simulink model "localization"  (R2025a)
settings: Solver=ode1  StartTime=0.0  StopTime=inf  FixedStep=1/60  RelTol=1e-3  EnableMultiTasking=on
model workspace (MAT data in the model file):
  downCamStepSize = Simulink.Parameter
  downCamStepSize.Value = Simulink.data.Expression
  downCamStepSize.Value.ExpressionString = "qc_get_step_size*ceil(1/60/qc_get_step_size)"
  downCamStepSize.Complexity = 'real'
  downCamStepSize.Dimensions = -1
  downCamStepSize.DataType = 'auto'
  lidarStepSize = Simulink.Parameter
  lidarStepSize.Value = Simulink.data.Expression
  lidarStepSize.Value.ExpressionString = "qc_get_step_size*ceil(1/5/qc_get_step_size)"
  lidarStepSize.Complexity = 'real'
  lidarStepSize.Dimensions = -1
  lidarStepSize.DataType = 'auto'
  mainStepSize = Simulink.Parameter
  mainStepSize.Value = Simulink.data.Expression
  mainStepSize.Value.ExpressionString = "qc_get_step_size"
  mainStepSize.Complexity = 'real'
  mainStepSize.Dimensions = -1
  mainStepSize.DataType = 'auto'
  mode = Simulink.Parameter
  mode.Value = 1
  mode.Complexity = 'real'
  mode.Dimensions = [1 1]
  mode.Description = '0 - education speeds via wheel speed commands
    | 1 - education speeds via body speed commands
    | 2 - research speeds via wheel speed commands
    | 3 - research speeds via body speed commands'
  mode.DataType = 'auto'
  realSenseStepSize = Simulink.Parameter
  realSenseStepSize.Value = Simulink.data.Expression
  realSenseStepSize.Value.ExpressionString = "qc_get_step_size*ceil(1/30/qc_get_step_size)"
  realSenseStepSize.Complexity = 'real'
  realSenseStepSize.Dimensions = -1
  realSenseStepSize.DataType = 'auto'
undefined symbols (not defined in the file): Point
libraries: quarc_library x17, simulink x1
settings Model: SimulationMode=external  ExtModeTrigDuration=10000  Creator=mbohra  LastModifiedBy=rdu
settings SolverCC: AlgebraicLoopSolver=TrustRegion  PositivePriorityOrder=on
settings DataIOCC: ReturnWorkspaceOutputs=off
settings DebuggingCC: ParameterPrecisionLossMsg=none  UnconnectedInputMsg=warning  UnconnectedOutputMsg=warning  UnconnectedLineMsg=warning  ArithmeticOperatorsInVariantConditions=warning
settings HardwareCC: ProdBitPerLong=64.0  ProdLargestAtomicInteger=LongLong  ProdLargestAtomicFloat=Double  ProdLongLongMode=on  ProdHWDeviceType=ARM Compatible->ARM 64-bit (LP64)
settings ModelReferenceCC: EnableRefExpFcnMdlSchedulingChecks=on
settings SFSimCC: SimUseLocalCustomCode=off  CustomCodeUndefinedFunction=UseInterfaceOnly
settings RTWCC: SystemTargetFile=quarc_linux_qbot_platform.tlc  TemplateMakefile=quarc_default_tmf  RTWUseLocalCustomCode=off  Toolchain=QUARC linux_qbot_platform | gmake (64-bit Windows)  BuildConfiguration=Faster Runs  GPUComputeCapability=3.5  Description=QUARC Linux QBot Platform Target Using Toolchain
settings CodeAppCC: StateflowObjectComments=on
settings STFCustomTargetCC: SystemTargetFile=quarc_linux_qbot_platform.tlc  TargetLangStandard=C99 (ISO)  MultiwordLength=2048.0  DynamicStringBufferSize=256.0  ConcurrentExecutionCompliant=on  UseToolchainInfoCompliant=on  MinimumThreadPriority=20.0  StripSymbols=off
settings GRTTargetCC: ExtMode=on  ExtModeMexFile=quarc_comm  ExtModeMexArgs='-w -d /tmp -uri %u','tcpip://192.168.5.4:17001'  ParMdlRefBuildCompliant=off  CompOptLevelCompliant=off  CombineOutputUpdateFcns=off  MatFileLogging=off  CPPClassGenCompliant=off  GRTInterface=on
settings ConfigComp: CovMetricSettings=dswe

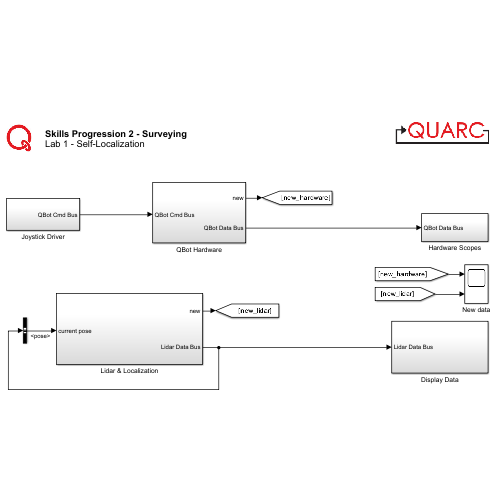
[thumbnail: Simulink's stored preview of the top-level diagram]
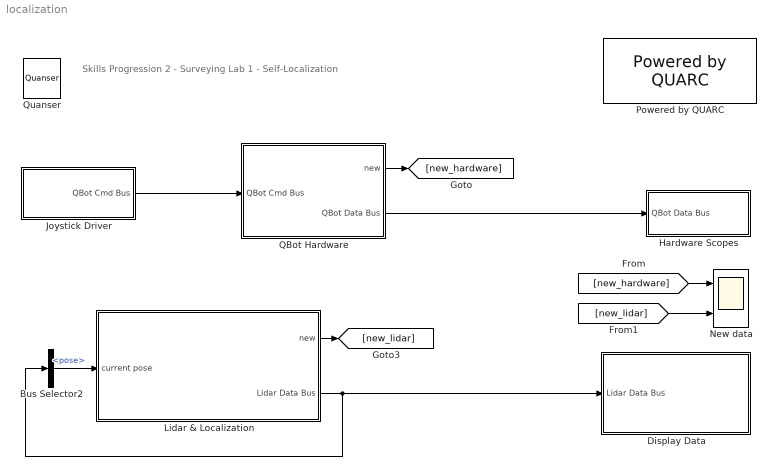
== system localization ==
  note: Skills Progression 2 - Surveying
      | Lab 1 - Self-Localization
  Bus Selector2 : BusSelector  OutputSignals=pose
  Display Data : Subsystem
  Hardware Scopes : Subsystem
  Joystick Driver : Subsystem
  Lidar & Localization : Subsystem
  New data : Scope  NumInputPorts=2
      settings: Title=Hardware Data New?  ActiveDisplayYMinimum=0.9  ActiveDisplayYMaximum=1.1  DataLoggingDecimation=10  DataLoggingVariableName=ScopeData2
  Powered by QUARC : quarc_library/Logos/Powered by QUARC
  QBot Hardware : Subsystem
  Quanser : quarc_library/Logos/Quanser
  wires:
  QBot Hardware/1(new) -> [new_hardware]
  Lidar & Localization/1(new) -> [new_lidar]
  [new_lidar] -> New data/2
  [new_hardware] -> New data/1
  Bus Selector2/1 -> Lidar & Localization/1(current pose)  "<pose>"
  Lidar & Localization/2(Lidar Data Bus) -> Bus Selector2/1, Display Data/1(Lidar Data Bus)
  Joystick Driver/1(QBot Cmd Bus) -> QBot Hardware/1(QBot Cmd Bus)
  QBot Hardware/2(QBot Data Bus) -> Hardware Scopes/1(QBot Data Bus)

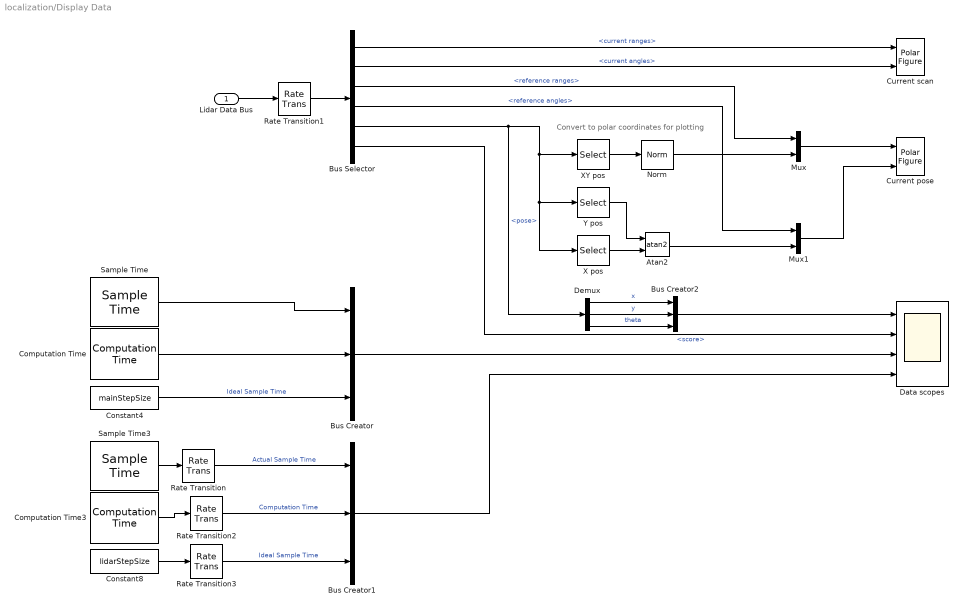
== system localization/Display Data ==
  note: Convert to polar coordinates for plotting
  Lidar Data Bus : Inport
  Atan2 : Trigonometry  Operator=atan2
  Bus Creator : BusCreator  Inputs=3
  Bus Creator1 : BusCreator  Inputs=3
  Bus Creator2 : BusCreator  Inputs=3
  Bus Selector : BusSelector  OutputSignals=current ranges,current angles,reference ranges,reference angles,pose,score
  Computation Time : quarc_library/Sources/Time/Computation Time  sample_time=mainStepSize  use_model=on  use_cpu_time=off
  Computation Time3 : quarc_library/Sources/Time/Computation Time  sample_time=lidarStepSize  use_model=on  use_cpu_time=off
  Constant4 : Constant  Value=mainStepSize
  Constant8 : Constant  Value=lidarStepSize
  Current pose : quarc_library/Sinks/Figures/Polar Figure  figure_mode=Use figure window  figure_tag=figure1  axes_tag=axes1  plot_mode=Frame-based  minimum_rho=0  maximum_rho=4  minimum_theta=0  maximum_theta=360  zero_location=right  direction=counterclockwise  buffer_size=421  update_rate=1  sample_time=-1  initial_position="875  207  831  654"  initial_visibility=off  line1_style=None  line1_width=0.5  line1_color=[1 0 0]  marker1=Point (.)  marker1_size=6  marker1_edge_color=[1 0 0]  marker1_face_color=[1 0 0]  line2_style=None  line2_width=0.5  line2_color=[0.85098 0.32549 0.0980392]  marker2=Cross (x)  marker2_size=6  marker2_edge_color=[0.85098 0.32549 0.0980392]  marker2_face_color=[0.85098 0.32549 0.0980392]  line3_style=Solid line (-)  line3_width=0.5  line3_color=[0.929412 0.694118 0.12549]  marker3=None  marker3_size=6  marker3_edge_color=[0.929412 0.694118 0.12549]  marker3_face_color=[0.929412 0.694118 0.12549]  line4_style=Solid line (-)  line4_width=0.5  line4_color=[0.494118 0.184314 0.556863]  marker4=None  marker4_size=6  marker4_edge_color=[0.494118 0.184314 0.556863]  marker4_face_color=[0.494118 0.184314 0.556863]  line5_style=Solid line (-)  line5_width=0.5  line5_color=[0.466667 0.67451 0.188235]  marker5=None  marker5_size=6  marker5_edge_color=[0.466667 0.67451 0.188235]  marker5_face_color=[0.466667 0.67451 0.188235]
      settings: SourceProductName=QUARC Targets
  Current scan : quarc_library/Sinks/Figures/Polar Figure  figure_mode=Use figure window  figure_tag=figure1  axes_tag=axes1  plot_mode=Frame-based  minimum_rho=0  maximum_rho=4  minimum_theta=0  maximum_theta=360  zero_location=right  direction=counterclockwise  buffer_size=2  update_rate=1  sample_time=-1  initial_position="60    84  1189   906"  initial_visibility=off  line1_style=None  line1_width=0.5  line1_color=[1 0 0]  marker1=Point (.)  marker1_size=6  marker1_edge_color=[1 0 0]  marker1_face_color=[1 0 0]  line2_style=Solid line (-)  line2_width=0.5  line2_color=[0.85098 0.32549 0.0980392]  marker2=None  marker2_size=6  marker2_edge_color=[0.85098 0.32549 0.0980392]  marker2_face_color=[0.85098 0.32549 0.0980392]  line3_style=Solid line (-)  line3_width=0.5  line3_color=[0.929412 0.694118 0.12549]  marker3=None  marker3_size=6  marker3_edge_color=[0.929412 0.694118 0.12549]  marker3_face_color=[0.929412 0.694118 0.12549]  line4_style=Solid line (-)  line4_width=0.5  line4_color=[0.494118 0.184314 0.556863]  marker4=None  marker4_size=6  marker4_edge_color=[0.494118 0.184314 0.556863]  marker4_face_color=[0.494118 0.184314 0.556863]  line5_style=Solid line (-)  line5_width=0.5  line5_color=[0.466667 0.67451 0.188235]  marker5=None  marker5_size=6  marker5_edge_color=[0.466667 0.67451 0.188235]  marker5_face_color=[0.466667 0.67451 0.188235]
      settings: SourceProductName=QUARC Targets
  Data scopes : Scope  NumInputPorts=4
      settings: ActiveDisplayString=4  Title=Lidar Timing  ActiveDisplayYMinimum=-0.063476284972040525  ActiveDisplayYMaximum=0.2359281248647544  DataLoggingDecimation=10  DataLoggingVariableName=ScopeData3
  Demux : Demux  Outputs=3
  Mux : Mux  Inputs=2
  Mux1 : Mux  Inputs=2
  Norm : quarc_library/Math Operations/Vectors/Norm
      settings: SourceProductName=QUARC Targets
  Rate Transition{,1..3} (4 alike) : RateTransition
  Sample Time : quarc_library/Sources/Time/Sample Time  Priority=-99  sample_time=mainStepSize
  Sample Time3 : quarc_library/Sources/Time/Sample Time  Priority=-99  sample_time=lidarStepSize
  X pos : Selector  InputPortWidth=3  IndexOptions=Index vector (dialog)  Indices=[1]  OutputSizes=1
  "XY pos " : Selector  InputPortWidth=3  IndexOptions=Index vector (dialog)  Indices=[1 2]  OutputSizes=1
  Y pos : Selector  InputPortWidth=3  IndexOptions=Index vector (dialog)  Indices=2  OutputSizes=1
  wires:
  Bus Selector/5 -> Demux/1, X pos/1, Y pos/1, "XY pos "/1  "<pose>"
  "XY pos "/1 -> Norm/1
  Y pos/1 -> Atan2/1
  X pos/1 -> Atan2/2
  Atan2/1 -> Mux1/2
  Norm/1 -> Mux/2
  Lidar Data Bus/1 -> Rate Transition1/1
  Bus Selector/1 -> Current scan/1  "<current ranges>"
  Bus Selector/2 -> Current scan/2  "<current angles>"
  Bus Selector/3 -> Mux/1  "<reference ranges>"
  Bus Selector/4 -> Mux1/1  "<reference angles>"
  Bus Selector/6 -> Data scopes/2  "<score>"
  Mux1/1 -> Current pose/2
  Mux/1 -> Current pose/1
  Sample Time3/1 -> Rate Transition/1
  Constant8/1 -> Rate Transition3/1
  Computation Time/1 -> Bus Creator/2
  Computation Time3/1 -> Rate Transition2/1
  Sample Time/1 -> Bus Creator/1
  Constant4/1 -> Bus Creator/3  "Ideal Sample Time"
  Rate Transition1/1 -> Bus Selector/1
  Bus Creator1/1 -> Data scopes/4
  Demux/1 -> Bus Creator2/1  "x"
  Demux/2 -> Bus Creator2/2  "y"
  Demux/3 -> Bus Creator2/3  "theta"
  Bus Creator2/1 -> Data scopes/1
  Rate Transition/1 -> Bus Creator1/1  "Actual Sample Time"
  Rate Transition2/1 -> Bus Creator1/2  "Computation Time"
  Rate Transition3/1 -> Bus Creator1/3  "Ideal Sample Time"
  Bus Creator/1 -> Data scopes/3

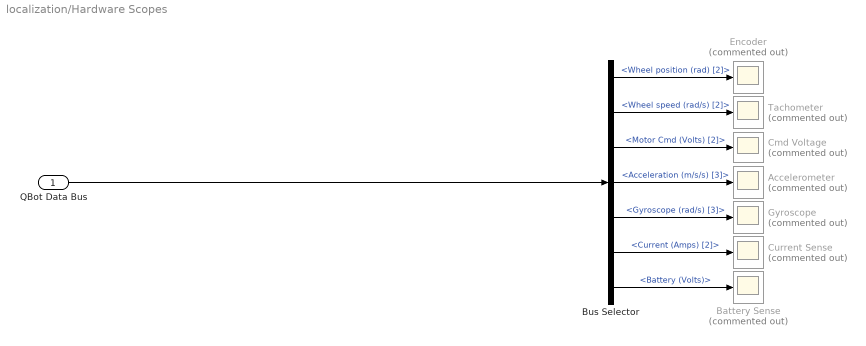
== system localization/Hardware Scopes ==
  QBot Data Bus : Inport
  Accelerometer : Scope  Commented=on
      settings: ActiveDisplayYMinimum=-1.32758  ActiveDisplayYMaximum=11.23  DataLoggingVariableName=ScopeData9
  Battery Sense : Scope  Commented=on
      settings: ActiveDisplayYMinimum=12.81161  ActiveDisplayYMaximum=12.96349  DataLoggingVariableName=ScopeData10
  Bus Selector : BusSelector  OutputSignals=Wheel position (rad) [2],Wheel speed (rad/s) [2],Motor Cmd (Volts) [2],Acceleration (m/s/s) [3],Gyroscope (rad/s) [3],Current (Amps) [2],Battery (Volts)
  Cmd Voltage : Scope  Commented=on
      settings: ActiveDisplayYMinimum=-1  ActiveDisplayYMaximum=1  DataLoggingVariableName=ScopeData11
  Current Sense : Scope  Commented=on
      settings: ActiveDisplayYMinimum=-0.05029  ActiveDisplayYMaximum=0.45265  DataLoggingVariableName=ScopeData12
  Encoder : Scope  Commented=on
      settings: ActiveDisplayYMinimum=-23.46955  ActiveDisplayYMaximum=23.65434  DataLoggingVariableName=ScopeData13
  Gyroscope : Scope  Commented=on
      settings: ActiveDisplayYMinimum=-0.40322  ActiveDisplayYMaximum=1.99912  DataLoggingVariableName=ScopeData14
  Tachometer : Scope  Commented=on
      settings: ActiveDisplayYMinimum=-11.69986  ActiveDisplayYMaximum=11.67552  DataLoggingVariableName=ScopeData15
  wires:
  Bus Selector/6 -> Current Sense/1  "<Current (Amps) [2]>"
  QBot Data Bus/1 -> Bus Selector/1
  Bus Selector/3 -> Cmd Voltage/1  "<Motor Cmd (Volts) [2]>"
  Bus Selector/7 -> Battery Sense/1  "<Battery (Volts)>"
  Bus Selector/4 -> Accelerometer/1  "<Acceleration (m/s/s) [3]>"
  Bus Selector/1 -> Encoder/1  "<Wheel position (rad) [2]>"
  Bus Selector/2 -> Tachometer/1  "<Wheel speed (rad/s) [2]>"
  Bus Selector/5 -> Gyroscope/1  "<Gyroscope (rad/s) [3]>"

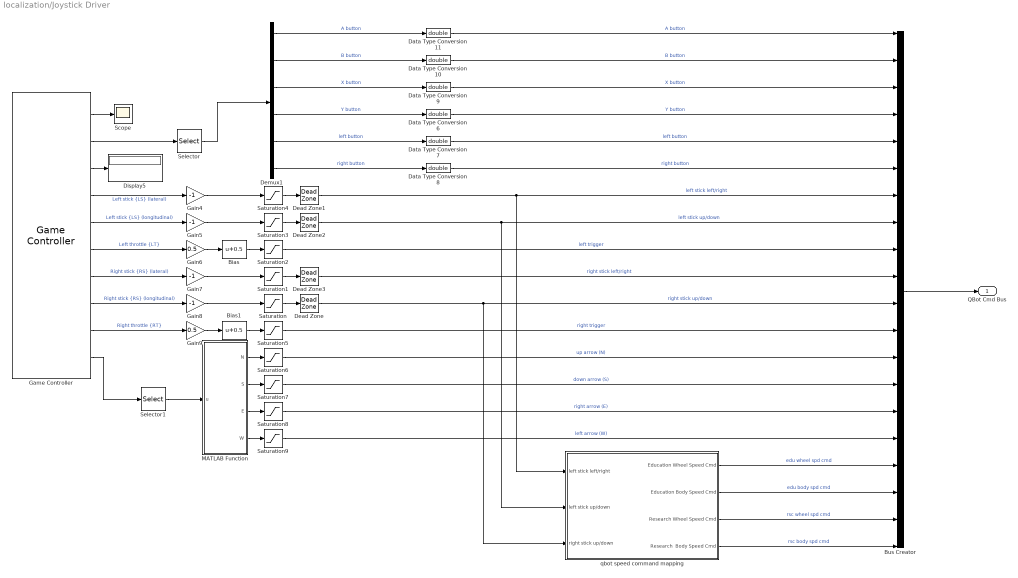
== system localization/Joystick Driver ==
  Bias : Bias  Bias=0.5  SaturateOnIntegerOverflow=off
  Bias1 : Bias  Bias=0.5  SaturateOnIntegerOverflow=off
  Bus Creator : BusCreator  Inputs=20
  Data Type Conversion{6..11} (6 alike) : DataTypeConversion  OutDataTypeStr=double  SaturateOnIntegerOverflow=off  RndMeth=Floor
  Dead Zone{,1..3} (4 alike) : DeadZone  LowerValue=-0.05  UpperValue=0.05
  Demux1 : Demux  Outputs=6
  Display5 : Display
  Gain{4..5,7..8} (4 alike) : Gain  Gain=-1
  Gain6 : Gain  Gain=0.5
  Gain9 : Gain  Gain=0.5
  Game Controller : quarc_library/Devices/Peripherals/Target/Game Controller  controller=1  buffer_size=12  deadzone=[]  saturation=[]  sample_time=qc_get_step_size  auto_center=off  enabled=on
      settings: SourceProductName=QUARC Targets
  MATLAB Function : MATLAB Function  TreatAsAtomicUnit=on
  Saturation{,1,3..4} (4 alike) : Saturate  UpperLimit=1  LowerLimit=-1
  Saturation{2,5..9} (6 alike) : Saturate  UpperLimit=1  LowerLimit=0
  Scope : Scope
      settings: ActiveDisplayYMinimum=-1  ActiveDisplayYMaximum=1
  Selector : Selector  InputPortWidth=32  IndexOptions=Index vector (dialog)  Indices=[1:6]  OutputSizes=1
  Selector1 : Selector  InputPortWidth=4  IndexOptions=Index vector (dialog)  Indices=1  OutputSizes=1
  qbot speed command mapping : Subsystem
  QBot Cmd Bus : Outport
  wires:
  Game Controller/1 -> Scope/1
  Game Controller/2 -> Selector/1
  Game Controller/3 -> Display5/1
  Game Controller/4 -> Gain4/1  "Left stick {LS} (lateral)"
  Game Controller/5 -> Gain5/1  "Left stick {LS} (longitudinal)"
  Game Controller/6 -> Gain6/1  "Left throttle {LT}"
  Game Controller/7 -> Gain7/1  "Right stick {RS} (lateral)"
  Game Controller/8 -> Gain8/1  "Right stick {RS} (longitudinal)"
  Game Controller/9 -> Gain9/1  "Right throttle {RT}"
  Game Controller/10 -> Selector1/1
  Selector/1 -> Demux1/1
  Selector1/1 -> MATLAB Function/1(u)
  Gain6/1 -> Bias/1
  Gain9/1 -> Bias1/1
  Gain8/1 -> Saturation/1
  Gain7/1 -> Saturation1/1
  Gain5/1 -> Saturation3/1
  Gain4/1 -> Saturation4/1
  Bias/1 -> Saturation2/1
  Bias1/1 -> Saturation5/1
  Saturation4/1 -> Dead Zone1/1
  Saturation3/1 -> Dead Zone2/1
  Saturation1/1 -> Dead Zone3/1
  Saturation/1 -> Dead Zone/1
  MATLAB Function/1(N) -> Saturation6/1
  MATLAB Function/2(S) -> Saturation7/1
  MATLAB Function/3(E) -> Saturation8/1
  MATLAB Function/4(W) -> Saturation9/1
  Demux1/5 -> Data Type Conversion7/1  "left button"
  Demux1/6 -> Data Type Conversion8/1  "right button"
  Dead Zone/1 -> qbot speed command mapping/3(right stick up/down), Bus Creator/11  "right stick up/down"
  Dead Zone1/1 -> qbot speed command mapping/1(left stick left/right), Bus Creator/7  "left stick left/right"
  Demux1/4 -> Data Type Conversion6/1  "Y button"
  Demux1/3 -> Data Type Conversion9/1  "X button"
  Demux1/2 -> Data Type Conversion10/1  "B button"
  Demux1/1 -> Data Type Conversion11/1  "A button"
  Dead Zone2/1 -> qbot speed command mapping/2(left stick up/down), Bus Creator/8  "left stick up/down"
  Saturation6/1 -> Bus Creator/13  "up arrow (N)"
  Saturation7/1 -> Bus Creator/14  "down arrow (S)"
  Saturation8/1 -> Bus Creator/15  "right arrow (E)"
  Saturation9/1 -> Bus Creator/16  "left arrow (W)"
  qbot speed command mapping/1(Education Wheel Speed Cmd) -> Bus Creator/17  "edu wheel spd cmd"
  qbot speed command mapping/2(Education Body Speed Cmd) -> Bus Creator/18  "edu body spd cmd"
  qbot speed command mapping/3(Research Wheel Speed Cmd) -> Bus Creator/19  "rsc wheel spd cmd"
  qbot speed command mapping/4(Research  Body Speed Cmd) -> Bus Creator/20  "rsc body spd cmd"
  Saturation2/1 -> Bus Creator/9  "left trigger"
  Dead Zone3/1 -> Bus Creator/10  "right stick left/right"
  Saturation5/1 -> Bus Creator/12  "right trigger"
  Bus Creator/1 -> QBot Cmd Bus/1
  Data Type Conversion6/1 -> Bus Creator/4  "Y button"
  Data Type Conversion8/1 -> Bus Creator/6  "right button"
  Data Type Conversion7/1 -> Bus Creator/5  "left button"
  Data Type Conversion9/1 -> Bus Creator/3  "X button"
  Data Type Conversion10/1 -> Bus Creator/2  "B button"
  Data Type Conversion11/1 -> Bus Creator/1  "A button"

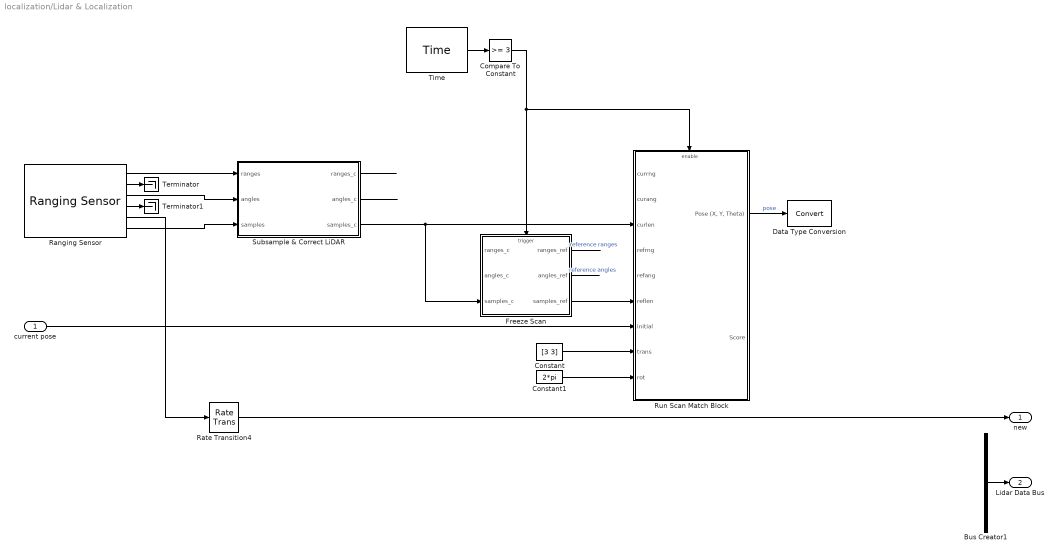
== system localization/Lidar & Localization ==
  current pose : Inport
  Bus Creator1 : BusCreator  Inputs=6
  Compare To Constant : simulink/Logic and Bit Operations/Compare To Constant  relop=>=  const=3  OutDataTypeStr=boolean
  Constant : Constant  Value=[3 3]
  Constant1 : Constant  Value=2*pi
  Data Type Conversion : DataTypeConversion  SaturateOnIntegerOverflow=off  RndMeth=Floor
  Freeze Scan : Subsystem  TreatAsAtomicUnit=on
  Ranging Sensor : quarc_library/Devices/Third-Party/Sensors/Ranging Sensor  sensor_type=Leishen M10P LIDAR  uri=serial://localhost:0?device='/dev/lidar',baud='512000',word='8',parity='none',stop='1',flow='none'  ranging_distance=Short  timing_budget=0.033  measurement_period=0.0005  output_mode=Fixed-size output  samples_per_revolution=1680  max_distance=0.050  max_angle=5  sample_time=lidarStepSize  show_versions=off  active=on
      settings: SourceProductName=QUARC Targets
  Rate Transition4 : RateTransition
  Run Scan Match Block : Subsystem
  Subsample & Correct LiDAR : Subsystem
  Terminator : Terminator
  Terminator1 : Terminator
  Time : quarc_library/Sources/Time/Time  time_source=Wall clock  sample_time=lidarStepSize
  new : Outport
  Lidar Data Bus : Outport  Port=2
  wires:
  Ranging Sensor/5 -> Rate Transition4/1
  Rate Transition4/1 -> new/1
  Ranging Sensor/2 -> Terminator/1
  Ranging Sensor/4 -> Terminator1/1
  Compare To Constant/1 -> Run Scan Match Block/Enable, Freeze Scan/Trigger
  Run Scan Match Block/1("Pose (X, Y, Theta)") -> Data Type Conversion/1  "pose"
  Freeze Scan/3(samples_ref) -> Run Scan Match Block/6(reflen)
  Time/1 -> Compare To Constant/1
  Bus Creator1/1 -> Lidar Data Bus/1
  current pose/1 -> Run Scan Match Block/7(initial)
  Constant/1 -> Run Scan Match Block/8(trans)
  Constant1/1 -> Run Scan Match Block/9(rot)
  Subsample & Correct LiDAR/3(samples_c) -> Freeze Scan/3(samples_c), Run Scan Match Block/3(curlen)
  Ranging Sensor/1 -> Subsample & Correct LiDAR/1(ranges)
  Ranging Sensor/3 -> Subsample & Correct LiDAR/2(angles)
  Ranging Sensor/6 -> Subsample & Correct LiDAR/3(samples)
  ? -> Freeze Scan/1(ranges_c)
  ? -> Freeze Scan/2(angles_c)
  Subsample & Correct LiDAR/1(ranges_c) -> ?
  Subsample & Correct LiDAR/2(angles_c) -> ?
  Freeze Scan/1(ranges_ref) -> ?  "reference ranges"
  Freeze Scan/2(angles_ref) -> ?  "reference angles"
  ? -> Bus Creator1/1  "current ranges"
  ? -> Bus Creator1/2  "current angles"
  ? -> Bus Creator1/3  "reference ranges"
  ? -> Bus Creator1/4  "reference angles"
  ? -> Bus Creator1/5  "pose"
  ? -> Bus Creator1/6  "score"

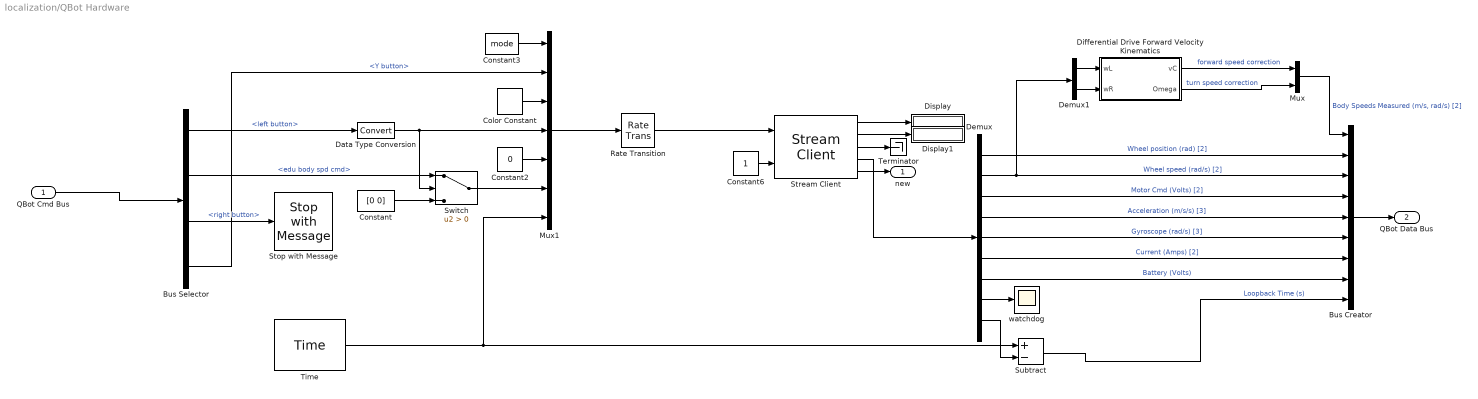
== system localization/QBot Hardware ==
  QBot Cmd Bus : Inport
  Bus Creator : BusCreator  Inputs=9
  Bus Selector : BusSelector  OutputSignals=left button,edu body spd cmd,right button,Y button
  Color Constant : quarc_library/Sources/Signals/Color Constant  color=[1 0 1]
      settings: SourceProductName=QUARC Targets
  Constant : Constant  Value=[0 0]
  Constant2 : Constant  Value=0
  Constant3 : Constant  Value=mode
  Constant6 : Constant
  Data Type Conversion : DataTypeConversion  SaturateOnIntegerOverflow=off  RndMeth=Floor
  Demux : Demux  Outputs=[2 2 2 3 3 2 1 1 1]
  Demux1 : Demux  Outputs=2
  Differential Drive Forward Velocity Kinematics : MATLAB Function  TreatAsAtomicUnit=on
  Display : Display
  Display1 : Display
  Mux : Mux  Inputs=2
  Mux1 : Mux  Inputs=7
  Rate Transition : RateTransition
  Stop with Message : quarc_library/Sinks/Error Handling/Stop with Message  message_type=Fixed error message  message_icon=Information  message=Operator: Emergency Stop
  Stream Client : quarc_library/Communications/Basic/Stream Client  uri_source=Specify via dialog (do not evaluate)  uri=tcpip://localhost:18888  send_buffer_size=1460  receive_buffer_size=1460  byte_order=little endian (Intel - LSB first)  optimization=Minimum latency  send_options=Send most recent data  receive_options=Receive most recent data  default_value=zeros(17,1)  sample_time=qc_get_step_size  active=off  implementation=Use blocking I/O in a separate thread  send_fifo_size=1000  receive_fifo_size=1000  send_priority=0  receive_priority=0  send_dimensions=off  receive_dimensions=off  max_dimensions=-1  data_type=Inherited via back propagation  type_expr=BusObject
      settings: AttributesFormatString="\"tcpip://localhost:18888\""
  Subtract : Sum  Inputs=+-
  Switch : Switch  Criteria=u2 > Threshold  SaturateOnIntegerOverflow=off  InputSameDT=off
  Terminator : Terminator
  Time : quarc_library/Sources/Time/Time  time_source=Wall clock  sample_time=qc_get_step_size
  watchdog : Scope
  new : Outport
  QBot Data Bus : Outport  Port=2
  wires:
  Constant3/1 -> Mux1/1
  Stream Client/3 -> Terminator/1
  Bus Selector/2 -> Switch/1  "<edu body spd cmd>"
  Stream Client/1 -> Display/1
  Constant6/1 -> Stream Client/2
  Stream Client/2 -> Display1/1
  Color Constant/1 -> Mux1/3
  Demux/3 -> Bus Creator/4  "Motor Cmd (Volts) [2]"
  Mux1/1 -> Rate Transition/1
  Stream Client/4 -> Demux/1
  Demux/1 -> Bus Creator/2  "Wheel position (rad) [2]"
  Stream Client/5 -> new/1
  Demux/7 -> Bus Creator/8  "Battery (Volts)"
  Demux/5 -> Bus Creator/6  "Gyroscope (rad/s) [3]"
  Demux/6 -> Bus Creator/7  "Current (Amps) [2]"
  Demux/9 -> Subtract/2
  Constant2/1 -> Mux1/5
  Demux/4 -> Bus Creator/5  "Acceleration (m/s/s) [3]"
  Time/1 -> Subtract/1, Mux1/7
  Bus Creator/1 -> QBot Data Bus/1
  Subtract/1 -> Bus Creator/9  "Loopback Time (s)"
  Demux/8 -> watchdog/1
  Switch/1 -> Mux1/6
  Constant/1 -> Switch/3
  QBot Cmd Bus/1 -> Bus Selector/1
  Bus Selector/3 -> Stop with Message/1  "<right button>"
  Bus Selector/1 -> Data Type Conversion/1  "<left button>"
  Data Type Conversion/1 -> Switch/2, Mux1/4
  Bus Selector/4 -> Mux1/2  "<Y button>"
  Demux/2 -> Bus Creator/3, Demux1/1  "Wheel speed (rad/s) [2]"
  Demux1/2 -> Differential Drive Forward Velocity Kinematics/2(wR)
  Demux1/1 -> Differential Drive Forward Velocity Kinematics/1(wL)
  Differential Drive Forward Velocity Kinematics/2(Omega) -> Mux/2  "turn speed correction"
  Differential Drive Forward Velocity Kinematics/1(vC) -> Mux/1  "forward speed correction"
  Mux/1 -> Bus Creator/1  "Body Speeds Measured (m/s, rad/s) [2]"
  Rate Transition/1 -> Stream Client/1

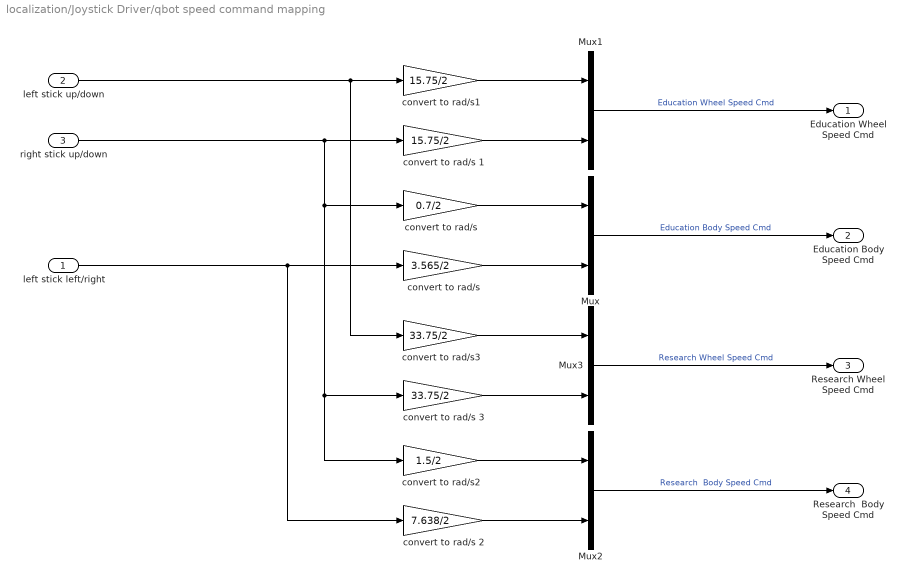
== system localization/Joystick Driver/qbot speed command mapping ==
  left stick left/right : Inport
  left stick up/down : Inport  Port=2
  right stick up/down : Inport  Port=3
  Mux{,1..3} (4 alike) : Mux  Inputs=2
  convert to rad/s : Gain  Gain=0.7/2
  "convert to rad/s " : Gain  Gain=3.565/2
  convert to rad/s 1 : Gain  Gain=15.75/2
  convert to rad/s 2 : Gain  Gain=7.638/2
  convert to rad/s 3 : Gain  Gain=33.75/2
  convert to rad/s1 : Gain  Gain=15.75/2
  convert to rad/s2 : Gain  Gain=1.5/2
  convert to rad/s3 : Gain  Gain=33.75/2
  Education Wheel Speed Cmd : Outport
  Education Body Speed Cmd : Outport  Port=2
  Research Wheel Speed Cmd : Outport  Port=3
  Research  Body Speed Cmd : Outport  Port=4
  wires:
  convert to rad/s/1 -> Mux/1
  Mux/1 -> Education Body Speed Cmd/1  "Education Body Speed Cmd"
  left stick left/right/1 -> convert to rad/s 2/1, "convert to rad/s "/1
  convert to rad/s2/1 -> Mux2/1
  left stick up/down/1 -> convert to rad/s3/1, convert to rad/s1/1
  right stick up/down/1 -> convert to rad/s 3/1, convert to rad/s2/1, convert to rad/s/1, convert to rad/s 1/1
  "convert to rad/s "/1 -> Mux/2
  convert to rad/s 3/1 -> Mux3/2
  convert to rad/s3/1 -> Mux3/1
  convert to rad/s 2/1 -> Mux2/2
  convert to rad/s 1/1 -> Mux1/2
  convert to rad/s1/1 -> Mux1/1
  Mux3/1 -> Research Wheel Speed Cmd/1  "Research Wheel Speed Cmd"
  Mux1/1 -> Education Wheel Speed Cmd/1  "Education Wheel Speed Cmd"
  Mux2/1 -> Research  Body Speed Cmd/1  "Research  Body Speed Cmd"

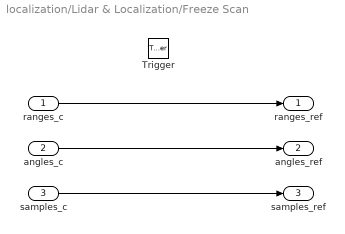
== system localization/Lidar & Localization/Freeze Scan ==
  ranges_c : Inport
  angles_c : Inport  Port=2
  samples_c : Inport  Port=3
  Trigger : TriggerPort  VariantControl=(inherit)  InitialTriggerSignalState=zero
  ranges_ref : Outport
  angles_ref : Outport  Port=2
  samples_ref : Outport  Port=3
  wires:
  ranges_c/1 -> ranges_ref/1
  angles_c/1 -> angles_ref/1
  samples_c/1 -> samples_ref/1

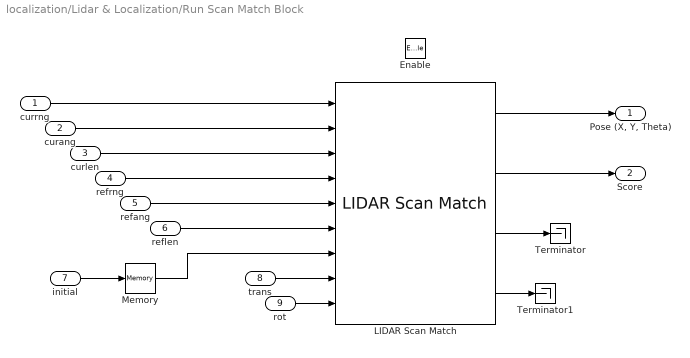
== system localization/Lidar & Localization/Run Scan Match Block ==
  currng : Inport
  curang : Inport  Port=2
  curlen : Inport  Port=3
  refrng : Inport  Port=4
  refang : Inport  Port=5
  reflen : Inport  Port=6
  initial : Inport  Port=7
  trans : Inport  Port=8
  rot : Inport  Port=9
  Enable : EnablePort
  LIDAR Scan Match : quarc_library/Image Processing/Generic/LIDAR Scan Match  mode=Fixed input with size  resolution=20  max_range=4  use_initial_pose=on
      settings: SourceProductName=QUARC Targets
  Memory : Memory  InitialCondition=[0 0 0]  InheritSampleTime=on
  Terminator : Terminator
  Terminator1 : Terminator
  "Pose (X, Y, Theta)" : Outport
  Score : Outport  Port=2
  wires:
  refrng/1 -> LIDAR Scan Match/4
  LIDAR Scan Match/2 -> Score/1
  curang/1 -> LIDAR Scan Match/2
  reflen/1 -> LIDAR Scan Match/6
  LIDAR Scan Match/1 -> "Pose (X, Y, Theta)"/1
  refang/1 -> LIDAR Scan Match/5
  currng/1 -> LIDAR Scan Match/1
  curlen/1 -> LIDAR Scan Match/3
  LIDAR Scan Match/3 -> Terminator/1
  LIDAR Scan Match/4 -> Terminator1/1
  Memory/1 -> LIDAR Scan Match/7
  initial/1 -> Memory/1
  trans/1 -> LIDAR Scan Match/8
  rot/1 -> LIDAR Scan Match/9

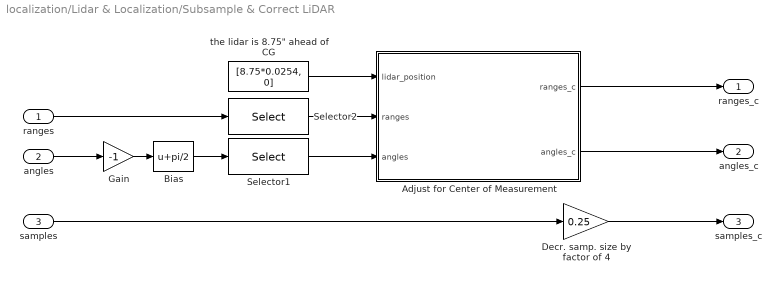
== system localization/Lidar & Localization/Subsample & Correct LiDAR ==
  ranges : Inport
  angles : Inport  Port=2
  samples : Inport  Port=3
  Adjust for Center of Measurement : MATLAB Function  TreatAsAtomicUnit=on  SystemSampleTime=lidarStepSize
  Bias : Bias  Bias=pi/2  SaturateOnIntegerOverflow=off
  "Decr. samp. size by factor of 4 " : Gain  Gain=0.25  OutDataTypeStr=int32
  Gain : Gain  Gain=-1
  Selector1 : Selector  InputPortWidth=1680  IndexOptions=Index vector (dialog)  Indices=[1:4:1677]  OutputSizes=1
  Selector2 : Selector  InputPortWidth=1680  IndexOptions=Index vector (dialog)  Indices=[1:4:1677]  OutputSizes=1
  "the lidar is 8.75\" ahead of CG" : Constant  Value=[8.75*0.0254, 0]  SampleTime=lidarStepSize
  ranges_c : Outport
  angles_c : Outport  Port=2
  samples_c : Outport  Port=3
  wires:
  Gain/1 -> Bias/1
  "the lidar is 8.75\" ahead of CG"/1 -> Adjust for Center of Measurement/1(lidar_position)
  samples/1 -> "Decr. samp. size by factor of 4 "/1
  Selector2/1 -> Adjust for Center of Measurement/2(ranges)
  Selector1/1 -> Adjust for Center of Measurement/3(angles)
  ranges/1 -> Selector2/1
  angles/1 -> Gain/1
  Bias/1 -> Selector1/1
  Adjust for Center of Measurement/1(ranges_c) -> ranges_c/1
  Adjust for Center of Measurement/2(angles_c) -> angles_c/1
  "Decr. samp. size by factor of 4 "/1 -> samples_c/1

== matlab function localization/Joystick Driver/MATLAB Function ==
  data: u input; N output; S output; E output; W output
function [N, S, E, W] = fcn(u)

N = 0;
S = 0;
E = 0;
W = 0;

switch u
    case 0
        N = 1;
    case 3.142
        S = 1;
    case 4.712
        W = 1;
    case 1.571
        E = 1;
    case 3.927
        S = 1;
        W = 1;
    case 2.356
        S = 1;
        E = 1;
    case 0.7854
        N = 1;
        E = 1;
    case 5.498
        N = 1;
        W = 1;
end

== matlab function localization/QBot Hardware/Differential Drive Forward Velocity Kinematics ==
  data: wL input; vC output; wR input; Omega output
function [vC , Omega] = forKin(wL, wR)

% calculate wheel angular velocities
wheelRadius = 3.5*0.0254/2;

vR = wR * wheelRadius;
vL = wL * wheelRadius;

% wheelbase
d=0.3928; 

% calculate wheel linear velocities
vC = (vR + vL)/2;
Omega = (vR - vL)/d;

== matlab function localization/Lidar & Localization/Subsample & Correct LiDAR/Adjust for Center of Measurement ==
  data: lidar_position input; ranges input; ranges_c output; angles input; angles_c output
function [ranges_c,angles_c] = correct_lidar(lidar_position, ranges,angles)

% Convert lidar data from polar into cartesian, and add lidar position
% Then Convert back into polar coordinates
%-------Replace the following line with your code---------%
ranges_c = ranges;
angles_c = angles./angles;
%---------------------------------------------------------%

end
